simulink model "state_space_all2"  (R2018a)
settings: Solver=FixedStepAuto  StartTime=0.0  StopTime=3  FixedStep=tm  MaxStep=1e-4  RelTol=1e-5  AbsTol=1e-5
InitFcn:
  | SimulinkInit_linea_transmision
values from neighbouring files (symbols this model uses):
  b = 4.91    [SimulinkInit_linea_transmision.m]
  C = 1    [SimulinkInit_linea_transmision.m]
  C1 = 22e-6    (= 2.2e-05)    [SimulinkInit_linea_transmision.m]
  C2 = 22e-6    (= 2.2e-05)    [SimulinkInit_linea_transmision.m]
  C3 = 610e-6    (= 0.00061)    [SimulinkInit_linea_transmision.m]
  Cl = 20000e-6    (= 0.02)    [SimulinkInit_linea_transmision.m]
  Jd = 0.3    [SimulinkInit_linea_transmision.m]
  K = 25    [SimulinkInit_linea_transmision.m]    (also in uio_linear.m = K1+E*H)
  K1 = 9.66    [SimulinkInit_linea_transmision.m]    (also in uio_linear.m = K1')
  K11 = 0.8    [SimulinkInit_linea_transmision.m]
  K1d = 1.15    [SimulinkInit_linea_transmision.m]
  K2 = 6.97    [SimulinkInit_linea_transmision.m]
  K22 = 0.2    [SimulinkInit_linea_transmision.m]
  K2d = 1    [SimulinkInit_linea_transmision.m]
  K3 = 31.8    [SimulinkInit_linea_transmision.m]
  K33 = 0.23    [SimulinkInit_linea_transmision.m]
  K3d = 1    [SimulinkInit_linea_transmision.m]
  K4 = 15.1    [SimulinkInit_linea_transmision.m]
  Kd = 0.02    [SimulinkInit_linea_transmision.m]
  Kdc = 0.02    [SimulinkInit_linea_transmision.m]
  Kf = 1    [SimulinkInit_linea_transmision.m]
  Kh = 1.2    [SimulinkInit_linea_transmision.m]
  Ks = 21.5    [SimulinkInit_linea_transmision.m]
  Ksc = 3    [SimulinkInit_linea_transmision.m]
  Kv = 1    [SimulinkInit_linea_transmision.m]
  L = 5.2    [SimulinkInit_linea_transmision.m]
  L1 = 40e-3    (= 0.04)    [SimulinkInit_linea_transmision.m]
  L2 = 30e-3    (= 0.03)    [SimulinkInit_linea_transmision.m]
  L3 = 5e-3    (= 0.005)    [SimulinkInit_linea_transmision.m]
  L4 = 35e-6    (= 3.5e-05)    [SimulinkInit_linea_transmision.m]
  L5 = 22e-6    (= 2.2e-05)    [SimulinkInit_linea_transmision.m]
  L6 = 10e-6    (= 1e-05)    [SimulinkInit_linea_transmision.m]
  Pd = 0.1    [SimulinkInit_linea_transmision.m]
  R = 10    [SimulinkInit_linea_transmision.m]
  R1 = 0.1    [SimulinkInit_linea_transmision.m]
  R2 = 0.2    [SimulinkInit_linea_transmision.m]
  R3 = 1e-3    (= 0.001)    [SimulinkInit_linea_transmision.m]
  R4 = 0.005    [SimulinkInit_linea_transmision.m]
  R5 = 0.0012    [SimulinkInit_linea_transmision.m]
  R6 = 0.001    [SimulinkInit_linea_transmision.m]
  RL = 10    [SimulinkInit_linea_transmision.m]
  Sbin = 13.8    [SimulinkInit_linea_transmision.m]
  Svin = 2.91    [SimulinkInit_linea_transmision.m]
  T1 = 0.4    [SimulinkInit_linea_transmision.m]
  T2 = 1    [SimulinkInit_linea_transmision.m]
  T3 = 15    [SimulinkInit_linea_transmision.m]
  T4 = 2.5    [SimulinkInit_linea_transmision.m]
  Tao1d = 0.5    [SimulinkInit_linea_transmision.m]
  Tao2d = 0.125    [SimulinkInit_linea_transmision.m]
  Tcd = 0.2    [SimulinkInit_linea_transmision.m]
  Tcr = 0.01    [SimulinkInit_linea_transmision.m]
  Tf = 0.04    [SimulinkInit_linea_transmision.m]
  Tr = 950    [SimulinkInit_linea_transmision.m]
  Tt = 450    [SimulinkInit_linea_transmision.m]
  Ttd = 0.04    [SimulinkInit_linea_transmision.m]
  Tv = 0.05    [SimulinkInit_linea_transmision.m]
  V = 20    [SimulinkInit_linea_transmision.m]
  wref = 70000    [SimulinkInit_linea_transmision.m]
  X_acid = 1.2    [SimulinkInit_linea_transmision.m]
  X_meth = 0.35    [SimulinkInit_linea_transmision.m]
  Z = 3    [SimulinkInit_linea_transmision.m]
undefined symbols (not defined in the file or in its folder): Ad, ataque, Bd, c11, c12, c13, c14, C1o, c21, c22, c23, c24, C2o, c31, c32, c33, c34, C3o, c41, c42, c43, c44, C4o, Cd, F1, F2, F3, F4, H1, H2, H3, H4, K1U, K2U, K3U, K4U, T1s, T2s, T3s, T4s, T5s, tao1, tao2, taod, tm
libraries: neural x277, dsparch4 x4, powerlib_meascontrol x4, mpclib x1, simulink x1
(part 6 of 15)

== system state_space_all2/Function Fitting Neural Network/Layer 2/Delays 1 ==
  "p{2}" : Inport  PortDimensions=30
      mask Display: e = 0.06;c1 = [120 230 180]/255;c2 = ([120 230 180]+0)/(256+128);c3 = ([120 230 180]+128)/(256+128);patch([0 1 1 0],[0 0 1 1],c1);patch([0 1 1 1-e 1-e 0+e],[0 0 1 1-e 0+e 0+e],c2);patch([0 0 1 1-e 0+e 0+e],[0 1 1 1-e 1-e 0+e],c3);plot([0 1 1 0 0],[0 0 1 1 0]);
  mux : Mux  Inputs=1
      mask Display: e = 0.06;c1 = [120 150 230]/255;c2 = ([120 150 230]+0)/383;c3 = ([120 150 230]+128)/383;patch([0 1 1 0],[0 0 1 1],c1);patch([0 1 1 1-e 1-e 0+e],[0 0 1 1-e 0+e 0+e],c2);patch([0 0 1 1-e 0+e 0+e],[0 1 1 1-e 1-e 0+e],c3);plot([0 1 1 0 0],[0 0 1 1 0]);disp('Mux')
  "pd{2,1}" : Outport
      mask Display: e = 0.06;c1 = [120 230 180]/255;c2 = ([120 230 180]+0)/(256+128);c3 = ([120 230 180]+128)/(256+128);patch([0 1 1 0],[0 0 1 1],c1);patch([0 1 1 1-e 1-e 0+e],[0 0 1 1-e 0+e 0+e],c2);patch([0 0 1 1-e 0+e 0+e],[0 1 1 1-e 1-e 0+e],c3);plot([0 1 1 0 0],[0 0 1 1 0]);
  wires:
  "p{2}"/1 -> mux/1
  mux/1 -> "pd{2,1}"/1

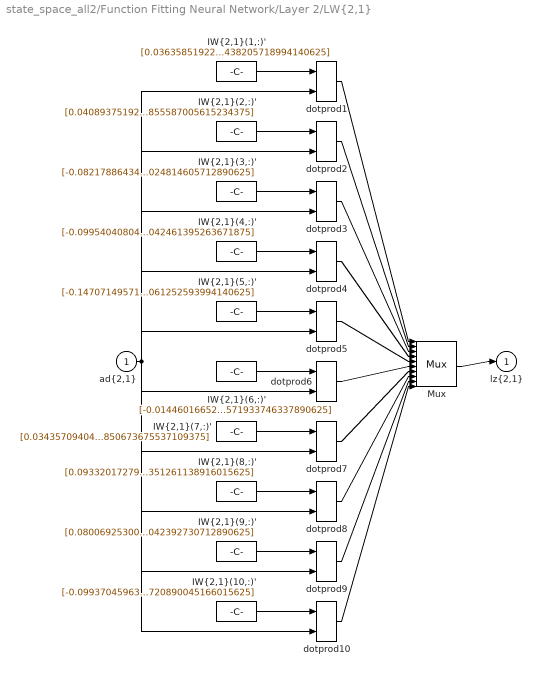
== system state_space_all2/Function Fitting Neural Network/Layer 2/LW{2,1} ==
  "ad{2,1}" : Inport  PortDimensions=30
      mask Display: e = 0.06;c1 = [120 230 180]/255;c2 = ([120 230 180]+0)/(256+128);c3 = ([120 230 180]+128)/(256+128);patch([0 1 1 0],[0 0 1 1],c1);patch([0 1 1 1-e 1-e 0+e],[0 0 1 1-e 0+e 0+e],c2);patch([0 0 1 1-e 0+e 0+e],[0 1 1 1-e 1-e 0+e],c3);plot([0 1 1 0 0],[0 0 1 1 0]);
  "IW{2,1}(1,:)'" : Constant  Value=[0.036358519226134956847662493828465812839567661285400390625;-0.01003690970632046229604750209318808629177510738372802734375;-0.1102332449938200620298545118203037418425083160400390625;-0.0770034337087573683700014726127847097814083099365234375;0.0237242544190229519285306736264828941784799098968505859375;0.07858299094587438415882019171476713381707668304443359375;0.0386784509914117891060669762737234123051166534423828125;0.04121133476905007586577056599708157591521739959716796875;-0.11394497686581379902737154452552204020321369171142578125;0.10349807460679701087702397899192874319851398468017578125;-0.0257970556152666737059764301420727861113846302032470703125;0.06729948029978470580569904768708511255681514739990234375;-0.0583071913875161940143954097948153503239154815673828125;-0.138612429594133501620234483198146335780620574951171875;0.10076275486304388240288432143643149174749851226806640625;-0.102565893483650694140152381805819459259510040283203125;-0.14195829636583312538533618862857110798358917236328125;-0.0519790953035916547531058995446073822677135467529296875;-0.0266688213459783385328449867301969788968563079833984375;0.0644213658467918948158370540113537572324275970458984375;-0.11399271172824702869075252920083585195243358612060546875;-0.042938885008907246021436776572954840958118438720703125;0.1532652704903950946491164586404920555651187896728515625;-0.03657741941101096128097225346209597773849964141845703125;-0.0028915150042861741640221051596881807199679315090179443359375;0.045183914187520747562931688889875658787786960601806640625;-0.036638891985520560812261692262836731970310211181640625;-0.1504555192101311167363064669189043343067169189453125;-0.1016757042015328516004757375412737019360065460205078125;-0.127027234678895484254468328799703158438205718994140625]
      mask Display: e = 0.06;c1 = [120 150 230]/255;c2 = ([120 150 230]+0)/383;c3 = ([120 150 230]+128)/383;patch([0 1 1 0],[0 0 1 1],c1);patch([0 1 1 1-e 1-e 0+e],[0 0 1 1-e 0+e 0+e],c2);patch([0 0 1 1-e 0+e 0+e],[0 1 1 1-e 1-e 0+e],c3);plot([0 1 1 0 0],[0 0 1 1 0]);disp('weights');
  "IW{2,1}(10,:)'" : Constant  Value=[-0.09937045963295616790578179688964155502617359161376953125;-0.052015401637255785638469518517013057135045528411865234375;0.2320308648477833746159859629187849350273609161376953125;0.2241408794756334643683004514969070442020893096923828125;0.05212955833449774145638144773329258896410465240478515625;-0.258946899579328537743805327409063465893268585205078125;-0.0165396484861428556822904312184618902392685413360595703125;-0.007641769084171921681825079275540701928548514842987060546875;-0.1302687365718275536163872629913385026156902313232421875;-0.0024510598281724592199803947067948683979921042919158935546875;-0.0280788792459086382347077659460410359315574169158935546875;0.143814450145818562010191499211941845715045928955078125;0.045713313246834426373244042451915447600185871124267578125;0.10488974243073180547813905150178470648825168609619140625;-0.137470216193598060439029495682916603982448577880859375;0.039462136151505060321920126398254069499671459197998046875;0.2116392145247512901473641022676019929349422454833984375;-0.079920111396243165291508603331749327480792999267578125;0.05782914857888458992629665544882300309836864471435546875;-0.2144427766412713987076443800106062553822994232177734375;0.036218992293589262476682932856419938616454601287841796875;-0.08381982570702406487583857597201131284236907958984375;-0.09810286412382918097563333503785543143749237060546875;0.253178191231142657446895327666425146162509918212890625;0.1820294983363882901361563426689826883375644683837890625;-0.10873768419112246619295802929627825506031513214111328125;0.045122707735696494790733623858614009805023670196533203125;0.059353541483675407997022688277866109274327754974365234375;0.09337888751986329893828298054359038360416889190673828125;0.014690295259942733052671570703751058317720890045166015625]
      mask Display: e = 0.06;c1 = [120 150 230]/255;c2 = ([120 150 230]+0)/383;c3 = ([120 150 230]+128)/383;patch([0 1 1 0],[0 0 1 1],c1);patch([0 1 1 1-e 1-e 0+e],[0 0 1 1-e 0+e 0+e],c2);patch([0 0 1 1-e 0+e 0+e],[0 1 1 1-e 1-e 0+e],c3);plot([0 1 1 0 0],[0 0 1 1 0]);disp('weights');
  "IW{2,1}(2,:)'" : Constant  Value=[0.040893751928160644582010974090735544450581073760986328125;0.019195412919876787827266895192224183119833469390869140625;-0.08004049542996662103266913845800445415079593658447265625;-0.06715891984862666641564743486014776863157749176025390625;-0.10336847574471604016554948657358181662857532501220703125;0.160654207973291607292054550271132029592990875244140625;-0.01538995857180412707432282104491605423390865325927734375;-0.00885792528196925089967184163697311305440962314605712890625;0.1500659094723615638589109266831655986607074737548828125;-0.0858031936156039287677543825338943861424922943115234375;0.0046174394283928950344364494640103657729923725128173828125;-0.1258493493776960125973829462964204140007495880126953125;0.09193367843333370703629014997204649262130260467529296875;-0.00949799799011893756961466550592376734130084514617919921875;0.067503092306094802932392440197872929275035858154296875;0.035937662854461961681185044881203793920576572418212890625;-0.049108171131423510036295709824116784147918224334716796875;0.1139195810272155828801743382427957840263843536376953125;-0.040179667035560438781427450294359005056321620941162109375;0.12460912207715772737071091569305281154811382293701171875;0.0851320971081593602658443842301494441926479339599609375;0.1031963872422962946728830502252094447612762451171875;-0.04100278808368985894450275964118191041052341461181640625;-0.1349446477806195698878610755855333991348743438720703125;-0.1499602172685186862732820145538426004350185394287109375;0.08380840466238483055239072427866631187498569488525390625;-0.010598397378240788369030411786297918297350406646728515625;0.039342354230936758818781839863731875084340572357177734375;0.00422333419072704226160386298261073534376919269561767578125;0.0884205938833347582228583405594690702855587005615234375]
      mask Display: e = 0.06;c1 = [120 150 230]/255;c2 = ([120 150 230]+0)/383;c3 = ([120 150 230]+128)/383;patch([0 1 1 0],[0 0 1 1],c1);patch([0 1 1 1-e 1-e 0+e],[0 0 1 1-e 0+e 0+e],c2);patch([0 0 1 1-e 0+e 0+e],[0 1 1 1-e 1-e 0+e],c3);plot([0 1 1 0 0],[0 0 1 1 0]);disp('weights');
  "IW{2,1}(3,:)'" : Constant  Value=[-0.08217886434204342560594369615500909276306629180908203125;0.1246010594062319787322934416806674562394618988037109375;0.052595984637784108650659931072368635796010494232177734375;0.225241289788105147895436175531358458101749420166015625;0.06591588057932930289073425456081167794764041900634765625;-0.01411758429810676569726712870078699779696762561798095703125;0.1706921552570712652396878183935768902301788330078125;-0.0620177326301019349319432194533874280750751495361328125;-0.211355875392802428081040488905273377895355224609375;0.00015409987467176824451307870500471608465886674821376800537109375;0.0304173977634369548106452185720627312548458576202392578125;0.2338477930004646265782497494001290760934352874755859375;0.1773732569917006729465214220908819697797298431396484375;-0.0959117398906082774256987022454268299043178558349609375;-0.0913603198477139499811272571605513803660869598388671875;-0.1764826723509100026010543160737142898142337799072265625;0.060150288375888261160895353896194137632846832275390625;0.053629892594864746191429816235540783964097499847412109375;0.06570634878028684677797599533732864074409008026123046875;0.03932115847319088419720145566316205076873302459716796875;0.16389657732019247138310902300872839987277984619140625;-0.139034548627867737824459481998928822576999664306640625;-0.09845239722023789441518459852886735461652278900146484375;0.03534297703585374816892539229229441843926906585693359375;0.004074170968328453233675556788284666254185140132904052734375;0.041339140945303047558478937162362853996455669403076171875;0.051401757629696821771947412571535096503794193267822265625;-0.1510897039995628687858442162905703298747539520263671875;-0.10761209115394614055372102257024380378425121307373046875;-0.043954093493524803992755778381251730024814605712890625]
      mask Display: e = 0.06;c1 = [120 150 230]/255;c2 = ([120 150 230]+0)/383;c3 = ([120 150 230]+128)/383;patch([0 1 1 0],[0 0 1 1],c1);patch([0 1 1 1-e 1-e 0+e],[0 0 1 1-e 0+e 0+e],c2);patch([0 0 1 1-e 0+e 0+e],[0 1 1 1-e 1-e 0+e],c3);plot([0 1 1 0 0],[0 0 1 1 0]);disp('weights');
  "IW{2,1}(4,:)'" : Constant  Value=[-0.09954040804320245239278364124402287416160106658935546875;0.045991204872785913793098444557472248561680316925048828125;-0.00518186792142237735714349611271245521493256092071533203125;0.0392040509757871913354421167241525836288928985595703125;0.2142957399217703395866152504822821356356143951416015625;-0.08723568954279026232967453324818052351474761962890625;0.044264767927613697662270197952238959260284900665283203125;0.06275045696450694265866587784330477006733417510986328125;-0.1331845726570379528919119138663518242537975311279296875;0.126546330022553998873036107397638261318206787109375;0.09625878679869249998635183374062762595713138580322265625;0.09759544881325778187264319285532110370695590972900390625;-0.172653211716482513082837613183073699474334716796875;-0.0095301764682810159723391763009203714318573474884033203125;-0.044378035250102983166886616572810453362762928009033203125;-0.1463649551927850012145171376687358133494853973388671875;-0.039303792662132928936724596269414178095757961273193359375;0.052061735408505858957450840307501493953168392181396484375;-0.11255209160717423444442175650692661292850971221923828125;-0.10184153319071707899379219952606945298612117767333984375;-0.06981071989202432270804621339266304858028888702392578125;-0.1607978897503663240353688479444826953113079071044921875;0.09768251131518086716187809770417516119778156280517578125;0.072902916094830405580040633140015415847301483154296875;-0.00700831509547000276738604185311487526632845401763916015625;-0.06856803410031449275141568477920372970402240753173828125;0.08838222744010783282764265322839492000639438629150390625;-0.1515340989006767336011449742727563716471195220947265625;-0.10015000503548247834384454790779273025691509246826171875;-0.15488686621895453310315815542708151042461395263671875]
      mask Display: e = 0.06;c1 = [120 150 230]/255;c2 = ([120 150 230]+0)/383;c3 = ([120 150 230]+128)/383;patch([0 1 1 0],[0 0 1 1],c1);patch([0 1 1 1-e 1-e 0+e],[0 0 1 1-e 0+e 0+e],c2);patch([0 0 1 1-e 0+e 0+e],[0 1 1 1-e 1-e 0+e],c3);plot([0 1 1 0 0],[0 0 1 1 0]);disp('weights');
  "IW{2,1}(5,:)'" : Constant  Value=[-0.1470714957178069770549200256937183439731597900390625;0.1594710056132574715892502581482403911650180816650390625;-0.0165584805104812445020190381228530895896255970001220703125;0.1007742013972511008201848881071782670915126800537109375;0.1103138175401983389622984077504952438175678253173828125;0.0650917234008910605691511364057078026235103607177734375;0.12221216293460966662021149886641069315373897552490234375;-0.00346520729717530832914018645851683686487376689910888671875;0.047174586405996705995580242642972734756767749786376953125;-0.0406575275120828749653156819476862438023090362548828125;0.175727921574451106945247147450572811067104339599609375;-0.041410483658788389826899134504856192506849765777587890625;0.07990653527085266050189460429464816115796566009521484375;0.01193503942972029031877045923693003715015947818756103515625;-0.1400968417910206376131299066400970332324504852294921875;-0.09596765691473761739072045884313411079347133636474609375;0.007263866531522889836980372280095252790488302707672119140625;0.289691673691975182247659859058330766856670379638671875;0.027804610518497828441919494935063994489610195159912109375;0.016979195500813455688149389288810198195278644561767578125;0.205289438488068298749311679785023443400859832763671875;-0.07588683555297172367293256911580101586878299713134765625;-0.06483996657338501889977777636886457912623882293701171875;-0.12886111390165744250424495476181618869304656982421875;-0.1765536799157837732909825945171178318560123443603515625;-0.032882605190245765836021263339716824702918529510498046875;0.16048260156357818662087311167852021753787994384765625;-0.022077407355061980098742679956558276899158954620361328125;-0.0841999662045012919886488589327200315892696380615234375;0.017724712755668538266551337301280000247061252593994140625]
      mask Display: e = 0.06;c1 = [120 150 230]/255;c2 = ([120 150 230]+0)/383;c3 = ([120 150 230]+128)/383;patch([0 1 1 0],[0 0 1 1],c1);patch([0 1 1 1-e 1-e 0+e],[0 0 1 1-e 0+e 0+e],c2);patch([0 0 1 1-e 0+e 0+e],[0 1 1 1-e 1-e 0+e],c3);plot([0 1 1 0 0],[0 0 1 1 0]);disp('weights');
  "IW{2,1}(6,:)'" : Constant  Value=[-0.0144601665232374776426382823046878911554813385009765625;-0.048839858552657912371675053009312250651419162750244140625;-0.054106993985066277608186879888307885266840457916259765625;-0.04496262089522122529228198573036934249103069305419921875;0.126942065303110529495000946553773246705532073974609375;-0.037163482911027841126827553352995892055332660675048828125;-0.026863739448628222439285906375516788102686405181884765625;0.0892496657558400074972126958527951501309871673583984375;-0.142128378974097191456138489229488186538219451904296875;0.1954538508130088114711497837561182677745819091796875;0.000251023855497998897058631317946719718747772276401519775390625;0.11400901812556864245440380045693018473684787750244140625;-0.2546241877256847363497627156903035938739776611328125;-0.06904533378620526795632628136445418931543827056884765625;0.110489904775116498658604768934310413897037506103515625;-0.06874590930524752951935596456678467802703380584716796875;-0.09443807611523570566536278647618019022047519683837890625;-0.04923614311127079423702213034630403853952884674072265625;-0.168652514586334623114538544541574083268642425537109375;-0.051728250990591029268017564390902407467365264892578125;-0.1655716241507886044015407378537929616868495941162109375;-0.0881897526365294226469160321357776410877704620361328125;0.2005664421013835518881052166761946864426136016845703125;0.060986761719255884461876604518693056888878345489501953125;0.058771667256910485599430415959432139061391353607177734375;-0.0283229019222654143650430569323361851274967193603515625;0.006221015678526447580110048107826514751650393009185791015625;-0.1161571080496283381311428684057318605482578277587890625;-0.06833176106146039707756045800124411471188068389892578125;-0.1850973848864942150616030858145677484571933746337890625]
      mask Display: e = 0.06;c1 = [120 150 230]/255;c2 = ([120 150 230]+0)/383;c3 = ([120 150 230]+128)/383;patch([0 1 1 0],[0 0 1 1],c1);patch([0 1 1 1-e 1-e 0+e],[0 0 1 1-e 0+e 0+e],c2);patch([0 0 1 1-e 0+e 0+e],[0 1 1 1-e 1-e 0+e],c3);plot([0 1 1 0 0],[0 0 1 1 0]);disp('weights');
  "IW{2,1}(7,:)'" : Constant  Value=[0.0343570940450702855262221646626130677759647369384765625;-0.102645026290050289663469129664008505642414093017578125;0.1199310290749309171332015466759912669658660888671875;0.055892981165330098136667658081933041103184223175048828125;-0.125094845545043187318157151821651495993137359619140625;-0.10140682787010520116144363100829650647938251495361328125;-0.090804481182373830705500949989072978496551513671875;0.00167717421208393897835708941101984237320721149444580078125;0.051663799572937492421420557775491033680737018585205078125;-0.10046585853196755844241039312692009843885898590087890625;-0.0943081393601929163228447805522591806948184967041015625;-0.031568418877034147562721244639760698191821575164794921875;0.06335071374960248025143272343484568409621715545654296875;0.09046792700835619427390810187716851942241191864013671875;-0.04008035284707982259799763369301217608153820037841796875;0.172148407258752189630257589669781737029552459716796875;0.1341191449218241960039676996530033648014068603515625;-0.09695624310024873737656747607616125606000423431396484375;0.10111895566917612765411860209496808238327503204345703125;-0.0605762592633916907569613385931006632745265960693359375;-0.0004759559412772511495515193047367574763484299182891845703125;0.08489774904560375146100881238453439436852931976318359375;-0.10674084865136156119458377133923931978642940521240234375;0.1354997101233960388189103696277015842497348785400390625;0.1352977911303644698026715786909335292875766754150390625;0.0065478582272752543225191601550250197760760784149169921875;-0.054826826293600972039854468675912357866764068603515625;0.1677587737984086724285504033105098642408847808837890625;0.157417126286422404124465401764609850943088531494140625;0.10934444574369671376867785284048295579850673675537109375]
      mask Display: e = 0.06;c1 = [120 150 230]/255;c2 = ([120 150 230]+0)/383;c3 = ([120 150 230]+128)/383;patch([0 1 1 0],[0 0 1 1],c1);patch([0 1 1 1-e 1-e 0+e],[0 0 1 1-e 0+e 0+e],c2);patch([0 0 1 1-e 0+e 0+e],[0 1 1 1-e 1-e 0+e],c3);plot([0 1 1 0 0],[0 0 1 1 0]);disp('weights');
  "IW{2,1}(8,:)'" : Constant  Value=[0.0933201727900848376773268455508514307439327239990234375;-0.0170408888059070291742802538692558300681412220001220703125;-0.08810513987667843716078408533576293848454952239990234375;-0.01114973710176687428374808774833581992425024509429931640625;-0.11111034605113108419960354922295664437115192413330078125;0.12785329733391470607983819718356244266033172607421875;0.0285207993099273367232360243406219524331390857696533203125;-0.01133624194106289638506179784371852292679250240325927734375;-0.136174622356371843867606230560340918600559234619140625;0.0231706525123088237505530884163817972876131534576416015625;-0.09291111419093149581538426673432695679366588592529296875;0.1134393440248903928146972930335323326289653778076171875;0.10113082204334265801204395529566681943833827972412109375;-0.1480799195461134643014844414210529066622257232666015625;0.117763109463666026943684528305311687290668487548828125;-0.068145389070960737942783680409775115549564361572265625;-0.0830497842344850856211024847652879543602466583251953125;-0.090280746636317521502945737665868364274501800537109375;0.06544762347768007249015909110312350094318389892578125;0.1274115127756960674787478637881577014923095703125;-0.039156928062962836900595675615477375686168670654296875;0.01221325559913450688187541715024053701199591159820556640625;0.0555036199501317550897283581434749066829681396484375;-0.054122953511469791554322483762007323093712329864501953125;0.0177693338248450620475704653244974906556308269500732421875;0.121266543241825563992364322984940372407436370849609375;-0.087846506476336239099822478237911127507686614990234375;-0.1133214007689109237286828602009336464107036590576171875;-0.0580237020303025208267655443705734796822071075439453125;-0.0697049576089877886975187948337406851351261138916015625]
      mask Display: e = 0.06;c1 = [120 150 230]/255;c2 = ([120 150 230]+0)/383;c3 = ([120 150 230]+128)/383;patch([0 1 1 0],[0 0 1 1],c1);patch([0 1 1 1-e 1-e 0+e],[0 0 1 1-e 0+e 0+e],c2);patch([0 0 1 1-e 0+e 0+e],[0 1 1 1-e 1-e 0+e],c3);plot([0 1 1 0 0],[0 0 1 1 0]);disp('weights');
  "IW{2,1}(9,:)'" : Constant  Value=[0.08006925300898208586186655111305299215018749237060546875;-0.0233719507985696121898921973070173407904803752899169921875;-0.047432198207011937174382154580598580650985240936279296875;0.0105288454990409598155398640528801479376852512359619140625;-0.09544052695661837948382100194066879339516162872314453125;0.06913762704131354297487632720731198787689208984375;0.035345147454833046596345269563244073651731014251708984375;-0.02282693916014377766288134807837195694446563720703125;-0.1467580180710079951200697223612223751842975616455078125;0.031891720120959921036529749471810646355152130126953125;-0.10346246016270888024024543483392335474491119384765625;0.1335561570860826219320216523556155152618885040283203125;0.0909584589730110248950722962035797536373138427734375;-0.1340928848983329313426793305552564561367034912109375;0.09735389736672865612643334998210775665938854217529296875;-0.0590605206794212189702619753006729297339916229248046875;-0.051361981686933531887628845424842438660562038421630859375;-0.12224373808665429941289204407439683564007282257080078125;0.0762213712955970290607865536003373563289642333984375;0.091778715459052528924388525410904549062252044677734375;-0.044678676478043667652517711985638015903532505035400390625;-0.00180404347308125013842061701296870523947291076183319091796875;0.03924944661939855361509899012162350118160247802734375;0.000645425075601213475706696698352970997802913188934326171875;0.058635002431721407190057249181336374022066593170166015625;0.09130831912835450647758506192985805682837963104248046875;-0.09080011525717703035898153984817327000200748443603515625;-0.10503198455027233648717555070106755010783672332763671875;-0.0423302229864706835993359845815575681626796722412109375;-0.059869228877928615251136079677962698042392730712890625]
      mask Display: e = 0.06;c1 = [120 150 230]/255;c2 = ([120 150 230]+0)/383;c3 = ([120 150 230]+128)/383;patch([0 1 1 0],[0 0 1 1],c1);patch([0 1 1 1-e 1-e 0+e],[0 0 1 1-e 0+e 0+e],c2);patch([0 0 1 1-e 0+e 0+e],[0 1 1 1-e 1-e 0+e],c3);plot([0 1 1 0 0],[0 0 1 1 0]);disp('weights');
  Mux : Mux  Inputs=10
      mask Display: e = 0.06;c1 = [120 150 230]/255;c2 = ([120 150 230]+0)/383;c3 = ([120 150 230]+128)/383;patch([0 1 1 0],[0 0 1 1],c1);patch([0 1 1 1-e 1-e 0+e],[0 0 1 1-e 0+e 0+e],c2);patch([0 0 1 1-e 0+e 0+e],[0 1 1 1-e 1-e 0+e],c3);plot([0 1 1 0 0],[0 0 1 1 0]);disp('Mux');
  dotprod{1..10} (10 alike) : neural/Weight Functions/dotprod
  "lz{2,1}" : Outport
      mask Display: e = 0.06;c1 = [120 230 180]/255;c2 = ([120 230 180]+0)/(256+128);c3 = ([120 230 180]+128)/(256+128);patch([0 1 1 0],[0 0 1 1],c1);patch([0 1 1 1-e 1-e 0+e],[0 0 1 1-e 0+e 0+e],c2);patch([0 0 1 1-e 0+e 0+e],[0 1 1 1-e 1-e 0+e],c3);plot([0 1 1 0 0],[0 0 1 1 0]);
  wires:
  "IW{2,1}(1,:)'"/1 -> dotprod1/1
  "ad{2,1}"/1 -> dotprod1/2, dotprod2/2, dotprod3/2, dotprod4/2, dotprod5/2, dotprod6/2, dotprod7/2, dotprod8/2, dotprod9/2, dotprod10/2
  dotprod1/1 -> Mux/1
  "IW{2,1}(2,:)'"/1 -> dotprod2/1
  dotprod2/1 -> Mux/2
  "IW{2,1}(3,:)'"/1 -> dotprod3/1
  dotprod3/1 -> Mux/3
  "IW{2,1}(4,:)'"/1 -> dotprod4/1
  dotprod4/1 -> Mux/4
  "IW{2,1}(5,:)'"/1 -> dotprod5/1
  dotprod5/1 -> Mux/5
  "IW{2,1}(6,:)'"/1 -> dotprod6/1
  dotprod6/1 -> Mux/6
  "IW{2,1}(7,:)'"/1 -> dotprod7/1
  dotprod7/1 -> Mux/7
  "IW{2,1}(8,:)'"/1 -> dotprod8/1
  dotprod8/1 -> Mux/8
  "IW{2,1}(9,:)'"/1 -> dotprod9/1
  dotprod9/1 -> Mux/9
  "IW{2,1}(10,:)'"/1 -> dotprod10/1
  dotprod10/1 -> Mux/10
  Mux/1 -> "lz{2,1}"/1

== system state_space_all2/Function Fitting Neural Network/Layer 3/Delays 1 ==
  "p{3}" : Inport  PortDimensions=10
      mask Display: e = 0.06;c1 = [120 230 180]/255;c2 = ([120 230 180]+0)/(256+128);c3 = ([120 230 180]+128)/(256+128);patch([0 1 1 0],[0 0 1 1],c1);patch([0 1 1 1-e 1-e 0+e],[0 0 1 1-e 0+e 0+e],c2);patch([0 0 1 1-e 0+e 0+e],[0 1 1 1-e 1-e 0+e],c3);plot([0 1 1 0 0],[0 0 1 1 0]);
  mux : Mux  Inputs=1
      mask Display: e = 0.06;c1 = [120 150 230]/255;c2 = ([120 150 230]+0)/383;c3 = ([120 150 230]+128)/383;patch([0 1 1 0],[0 0 1 1],c1);patch([0 1 1 1-e 1-e 0+e],[0 0 1 1-e 0+e 0+e],c2);patch([0 0 1 1-e 0+e 0+e],[0 1 1 1-e 1-e 0+e],c3);plot([0 1 1 0 0],[0 0 1 1 0]);disp('Mux')
  "pd{3,2}" : Outport
      mask Display: e = 0.06;c1 = [120 230 180]/255;c2 = ([120 230 180]+0)/(256+128);c3 = ([120 230 180]+128)/(256+128);patch([0 1 1 0],[0 0 1 1],c1);patch([0 1 1 1-e 1-e 0+e],[0 0 1 1-e 0+e 0+e],c2);patch([0 0 1 1-e 0+e 0+e],[0 1 1 1-e 1-e 0+e],c3);plot([0 1 1 0 0],[0 0 1 1 0]);
  wires:
  "p{3}"/1 -> mux/1
  mux/1 -> "pd{3,2}"/1

== system state_space_all2/Function Fitting Neural Network/Layer 3/LW{3,2} ==
  "ad{3,2}" : Inport  PortDimensions=10
      mask Display: e = 0.06;c1 = [120 230 180]/255;c2 = ([120 230 180]+0)/(256+128);c3 = ([120 230 180]+128)/(256+128);patch([0 1 1 0],[0 0 1 1],c1);patch([0 1 1 1-e 1-e 0+e],[0 0 1 1-e 0+e 0+e],c2);patch([0 0 1 1-e 0+e 0+e],[0 1 1 1-e 1-e 0+e],c3);plot([0 1 1 0 0],[0 0 1 1 0]);
  "IW{3,2}(1,:)'" : Constant  Value=[0.2489725454796852532890483189476071856915950775146484375;0.32771438331702762436492548658861778676509857177734375;0.345975470038703047936934353856486268341541290283203125;-0.2931596291362199568908408764400519430637359619140625;-0.07885416518131395380297732344843097962439060211181640625;-0.305290044297352014535107400661217980086803436279296875;-0.1878819984156337163927474875890766270458698272705078125;0.5267133307651270524019082586164586246013641357421875;0.4660108224317813796488962907460518181324005126953125;-0.3701322421960469011281702478299848735332489013671875]
      mask Display: e = 0.06;c1 = [120 150 230]/255;c2 = ([120 150 230]+0)/383;c3 = ([120 150 230]+128)/383;patch([0 1 1 0],[0 0 1 1],c1);patch([0 1 1 1-e 1-e 0+e],[0 0 1 1-e 0+e 0+e],c2);patch([0 0 1 1-e 0+e 0+e],[0 1 1 1-e 1-e 0+e],c3);plot([0 1 1 0 0],[0 0 1 1 0]);disp('weights');
  "IW{3,2}(2,:)'" : Constant  Value=[0.278150783315833260989080599756562151014804840087890625;0.394592664448457253190127858033520169556140899658203125;-0.390386884407995793377921245337347500026226043701171875;-0.0530760947044109643311315949176787398755550384521484375;-0.035429047900210820787325616265661665238440036773681640625;0.13058175988364506547867449626210145652294158935546875;-0.383398266142291610503178844737703911960124969482421875;0.16267799718867459457527502308948896825313568115234375;0.023410566368326911346198215824188082478940486907958984375;-0.73719966967300043503286133272922597825527191162109375]
      mask Display: e = 0.06;c1 = [120 150 230]/255;c2 = ([120 150 230]+0)/383;c3 = ([120 150 230]+128)/383;patch([0 1 1 0],[0 0 1 1],c1);patch([0 1 1 1-e 1-e 0+e],[0 0 1 1-e 0+e 0+e],c2);patch([0 0 1 1-e 0+e 0+e],[0 1 1 1-e 1-e 0+e],c3);plot([0 1 1 0 0],[0 0 1 1 0]);disp('weights');
  "IW{3,2}(3,:)'" : Constant  Value=[0.6462446177559417748170744744129478931427001953125;-0.357765293637721359942815979593433439731597900390625;0.400709104168131935441721225288347341120243072509765625;0.8278029938403783649647493803058750927448272705078125;-0.10681415197411105177938139831894659437239170074462890625;0.85346283553546908873244092319509945809841156005859375;-0.477839509821052388360840268433094024658203125;0.2660563174762209381896127524669282138347625732421875;0.294146378216100401470356473510037176311016082763671875;-0.011172859304117994938554403461239417083561420440673828125]
      mask Display: e = 0.06;c1 = [120 150 230]/255;c2 = ([120 150 230]+0)/383;c3 = ([120 150 230]+128)/383;patch([0 1 1 0],[0 0 1 1],c1);patch([0 1 1 1-e 1-e 0+e],[0 0 1 1-e 0+e 0+e],c2);patch([0 0 1 1-e 0+e 0+e],[0 1 1 1-e 1-e 0+e],c3);plot([0 1 1 0 0],[0 0 1 1 0]);disp('weights');
  "IW{3,2}(4,:)'" : Constant  Value=[0.2099288087752183284973028776221326552331447601318359375;-0.129963658657175351596180234992061741650104522705078125;-0.6516734655383895624680690161767415702342987060546875;-0.320391831798870374559129459157702513039112091064453125;-0.90469492447328125894756567504373379051685333251953125;0.29933618118387206319397364495671354234218597412109375;0.54312963811024606020083638213691301643848419189453125;0.296201286702774069237165122103760950267314910888671875;0.35172962715573341530017614786629565060138702392578125;0.0674961321208523978842919177623116411268711090087890625]
      mask Display: e = 0.06;c1 = [120 150 230]/255;c2 = ([120 150 230]+0)/383;c3 = ([120 150 230]+128)/383;patch([0 1 1 0],[0 0 1 1],c1);patch([0 1 1 1-e 1-e 0+e],[0 0 1 1-e 0+e 0+e],c2);patch([0 0 1 1-e 0+e 0+e],[0 1 1 1-e 1-e 0+e],c3);plot([0 1 1 0 0],[0 0 1 1 0]);disp('weights');
  Mux : Mux
      mask Display: e = 0.06;c1 = [120 150 230]/255;c2 = ([120 150 230]+0)/383;c3 = ([120 150 230]+128)/383;patch([0 1 1 0],[0 0 1 1],c1);patch([0 1 1 1-e 1-e 0+e],[0 0 1 1-e 0+e 0+e],c2);patch([0 0 1 1-e 0+e 0+e],[0 1 1 1-e 1-e 0+e],c3);plot([0 1 1 0 0],[0 0 1 1 0]);disp('Mux');
  dotprod{1..4} (4 alike) : neural/Weight Functions/dotprod
  "lz{3,2}" : Outport
      mask Display: e = 0.06;c1 = [120 230 180]/255;c2 = ([120 230 180]+0)/(256+128);c3 = ([120 230 180]+128)/(256+128);patch([0 1 1 0],[0 0 1 1],c1);patch([0 1 1 1-e 1-e 0+e],[0 0 1 1-e 0+e 0+e],c2);patch([0 0 1 1-e 0+e 0+e],[0 1 1 1-e 1-e 0+e],c3);plot([0 1 1 0 0],[0 0 1 1 0]);
  wires:
  "IW{3,2}(1,:)'"/1 -> dotprod1/1
  "ad{3,2}"/1 -> dotprod1/2, dotprod2/2, dotprod3/2, dotprod4/2
  dotprod1/1 -> Mux/1
  "IW{3,2}(2,:)'"/1 -> dotprod2/1
  dotprod2/1 -> Mux/2
  "IW{3,2}(3,:)'"/1 -> dotprod3/1
  dotprod3/1 -> Mux/3
  "IW{3,2}(4,:)'"/1 -> dotprod4/1
  dotprod4/1 -> Mux/4
  Mux/1 -> "lz{3,2}"/1

== system state_space_all2/Function Fitting Neural Network1/Layer 1/Delays 1 ==
  "p{1}" : Inport  PortDimensions=44  SampleTime=4e-05
      mask Display: e = 0.06;c1 = [120 230 180]/255;c2 = ([120 230 180]+0)/(256+128);c3 = ([120 230 180]+128)/(256+128);patch([0 1 1 0],[0 0 1 1],c1);patch([0 1 1 1-e 1-e 0+e],[0 0 1 1-e 0+e 0+e],c2);patch([0 0 1 1-e 0+e 0+e],[0 1 1 1-e 1-e 0+e],c3);plot([0 1 1 0 0],[0 0 1 1 0]);
  mux : Mux  Inputs=1
      mask Display: e = 0.06;c1 = [120 150 230]/255;c2 = ([120 150 230]+0)/383;c3 = ([120 150 230]+128)/383;patch([0 1 1 0],[0 0 1 1],c1);patch([0 1 1 1-e 1-e 0+e],[0 0 1 1-e 0+e 0+e],c2);patch([0 0 1 1-e 0+e 0+e],[0 1 1 1-e 1-e 0+e],c3);plot([0 1 1 0 0],[0 0 1 1 0]);disp('Mux')
  "pd{1,1}" : Outport
      mask Display: e = 0.06;c1 = [120 230 180]/255;c2 = ([120 230 180]+0)/(256+128);c3 = ([120 230 180]+128)/(256+128);patch([0 1 1 0],[0 0 1 1],c1);patch([0 1 1 1-e 1-e 0+e],[0 0 1 1-e 0+e 0+e],c2);patch([0 0 1 1-e 0+e 0+e],[0 1 1 1-e 1-e 0+e],c3);plot([0 1 1 0 0],[0 0 1 1 0]);
  wires:
  "p{1}"/1 -> mux/1
  mux/1 -> "pd{1,1}"/1
